simulink library "xblocks_library_pfbs"  (Simulink 7.6)
settings: Solver=ode45  SolverMode=SingleTasking  StartTime=0.0  StopTime=10.0  RelTol=1e-3
libraries: xbsIndex_r4 x369, monroe_library x47
(part 3 of 7)

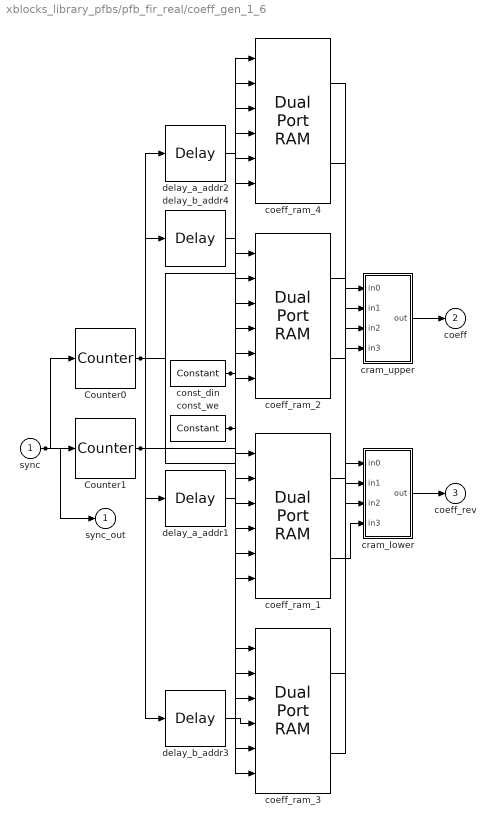
== system xblocks_library_pfbs/pfb_fir_real/coeff_gen_1_6 ==
  sync : Inport
  Counter0 : xbsIndex_r4/Counter  cnt_type=Free Running  cnt_to=Inf  operation=Up  start_count=8  cnt_by_val=1  arith_type=Unsigned  n_bits=11  bin_pt=0  load_pin=off  rst=on  en=off  explicit_period=on  period=1  dbl_ovrd=off  use_behavioral_HDL=off  implementation=Fabric  block_type=counter
  Counter1 : xbsIndex_r4/Counter  cnt_type=Free Running  cnt_to=Inf  operation=Down  start_count=2039  cnt_by_val=1  arith_type=Unsigned  n_bits=11  bin_pt=0  load_pin=off  rst=on  en=off  explicit_period=on  period=1  dbl_ovrd=off  use_behavioral_HDL=off  implementation=Fabric  block_type=counter
  coeff_ram_1 : xbsIndex_r4/Dual Port RAM  depth=2048  initVector=[-3.66227706703549e-006 -2.32001223055732e-005 -4.27476852292724e-005 -6.23051253222115e-005 -8.1872602220841e-005 -0.000101450275712516 -0.000121038305734028 -0.000140636852370183 -0.00016024607585228 -0.000179866136556684 -0.000199497195003349 -0.000219139411854352 -0.000238792947912406 -0.000258457964119436 -0.000278134621555034 -0.000297823081435025 -0.00031752350510998 -0.000337236054063722 -0.000356960889911885 -0.000376698174400365 -0.000396448069403875 -0.000416210736924445 -0.000435986339089932 -0.000455775038152512 -0.000475576996487234 -0.000495392376590451 -0.000515221341078369 -0.000535064052685532 -0.000554920674263309 -0.000574791368778434 -0.000594676299311432 -0.000614575629055151 -0.000634489521313247 -0.000654418139498664 -0.000674361647132113 -0.000694320207840599 -0.000714293985355835 -0.000734283143512765 -0.000754287846248034 -0.000774308257598449 -0.000794344541699504 -0.000814396862783775 -0.000834465385179446 -0.00085455027330876 -0.000874651691686487 -0.000894769804918378 -0.000914904777699676 -0.000935056774813504 -0.000955225961129376 -0.000975412501601635 -0.00099561656126791 -0.00101583830524761 -0.00103607789874029 -0.00105633550702419 -0.00107661129545462 -0.00109690542946247 -0.00111721807455258 -0.00113754939630225 -0.00115789956035966 -0.00117826873244228 -0.00119865707833536 -0.00121906476389031 -0.00123949195502323 -0.00125993881771322 -0.00128040551800089 -0.00130089222198679 -0.00132139909582981 -0.00134192630574561 -0.00136247401800508 -0.00138304239893273 -0.0014036316149051 -0.00142424183234923 -0.00144487321774102 -0.00146552593760373 -0.0014862001585063 -0.00150689604706182 -0.00152761376992592 -0.00154835349379522 -0.00156911538540568 -0.00158989961153107 -0.00161070633898134 -0.00163153573460101 -0.00165238796526762 -0.00167326319789008 -0.00169416159940713 -0.00171508333678569 -0.00173602857701927 -0.00175699748712639 -0.00177799023414891 -0.00179900698515051 -0.00182004790721505 -0.0018411131674449 -0.00186220293295942 -0.00188331737089327 -0.00190445664839487 -0.00192562093262472 -0.00194681039075383 -0.00196802518996205 -0.00198926549743652 -0.00201053148036997 -0.00203182330595915 -0.00205314114140324 -0.0020744851539021 -0.00209585551065479 -0.00211725237885783 -0.00213867592570362 -0.00216012631837886 -0.00218160372406278 -0.00220310830992565 -0.00222464024312707 -0.00224619969081432 -0.00226778682012079 -0.00228940179816431 -0.00231104479204548 -0.00233271596884606 -0.00235441549562733 -0.00237614353942842 -0.00239790026726473 -0.00241968584612619 -0.0024415004429757 -0.00246334422474741 -0.00248521735834514 -0.00250712001064065 -0.0025290523484721 -0.00255101453864227 -0.00257300674791699 -0.00259502914302347 -0.00261708189064861 -0.0026391651574374 -0.00266127910999121 -0.00268342391486616 -0.00270559973857143 -0.00272780674756764 -0.00275004510826513 -0.0027723149870224 -0.00279461655014431 -0.00281694996388051 -0.00283931539442373 -0.00286171300790811 -0.0028841429704076 -0.00290660544793418 -0.00292910060643627 -0.00295162861179701 -0.00297418962983265 -0.00299678382629077 -0.00301941136684874 -0.00304207241711193 -0.00306476714261208 -0.00308749570880561 -0.00311025828107197 -0.00313305502471193 -0.0031558861049459 -0.00317875168691227 -0.00320165193566569 -0.00322458701617542 -0.00324755709332363 -0.00327056233190375 -0.00329360289661871 -0.00331667895207931 -0.00333979066280252 -0.00336293819320978 -0.00338612170762535 -0.00340934137027454 -0.0034325973452821 -0.00345588979667048 -0.00347921888835816 -0.00350258478415793 -0.00352598764777525 -0.00354942764280647 -0.00357290493273721 -0.00359641968094064 -0.00361997205067573 -0.00364356220508568 -0.00366719030719606 -0.00369085651991323 -0.00371456100602259 -0.00373830392818688 -0.00376208544894448 -0.00378590573070776 -0.00380976493576126 -0.0038336632262601 -0.00385760076422821 -0.00388157771155665 -0.00390559423000192 -0.00392965048118421 -0.0039537466265857 -0.0039778828275489 -0.0040020592452749 ...(+37226 chars)]  distributed_mem=Block RAM  init_a=0  init_b=0  rst_a=off  rst_b=off  en_a=off  en_b=off  latency=2  write_mode_A=No Read On Write  write_mode_B=No Read On Write  dbl_ovrd=off  optimize=Area  use_rpm=on  block_type=dpram
  coeff_ram_2 : xbsIndex_r4/Dual Port RAM  depth=2048  initVector=[4.94480501293789e-005 0.000313528515560473 0.000578211328821063 0.000843496748818215 0.00110938503293764 0.00137587643704166 0.00164297121546728 0.00191066962102343 0.00217897190498901 0.00244787831711094 0.00271738910560136 0.00298750451713606 0.00325822479685175 0.0035295501883441 0.00380148093366576 0.00407401727332372 0.00434715944627736 0.00462090768993652 0.00489526224015883 0.00517022333124779 0.00544579119595085 0.00572196606545669 0.00599874816939369 0.00627613773582724 0.00655413499125781 0.00683274016061908 0.00711195346727528 0.00739177513301934 0.00767220537807098 0.00795324442107411 0.00823489247909495 0.00851714976762013 0.0088000165005541 0.00908349289021755 0.00936757914734485 0.00965227548108216 0.00993758209898553 0.0102234992070184 0.0105100270095498 0.0107971657093523 0.0110849155075997 0.0113732766038651 0.0116622491961191 0.0119518334807271 0.012242029652448 0.0125328379044316 0.0128242584282165 0.0131162914137289 0.0134089370492794 0.0137021955215617 0.0139960670156506 0.0142905517149995 0.0145856498014388 0.014881361455174 0.0151776868547828 0.0154746261772146 0.015772179597787 0.0160703472901847 0.0163691294264574 0.0166685261770175 0.0169685377106383 0.0172691641944524 0.0175704057939489 0.0178722626729722 0.0181747349937197 0.01847782291674 0.0187815266009308 0.019085846203537 0.0193907818801487 0.0196963337846997 0.0200025020694647 0.0203092868850582 0.0206166883804326 0.0209247067028753 0.0212333419980079 0.0215425944097839 0.0218524640804866 0.0221629511507274 0.0224740557594439 0.0227857780438981 0.0230981181396744 0.0234110761806776 0.0237246522991314 0.0240388466255762 0.0243536592888676 0.0246690904161739 0.0249851401329752 0.0253018085630606 0.0256190958285271 0.0259370020497773 0.0262555273455178 0.0265746718327575 0.0268944356268053 0.0272148188412687 0.0275358215880523 0.0278574439773549 0.028179686117669 0.0285025481157782 0.0288260300767556 0.0291501321039621 0.0294748542990447 0.0298001967619343 0.0301261595908447 0.0304527428822702 0.0307799467309838 0.0311077712300362 0.0314362164707532 0.0317652825427343 0.0320949695338515 0.0324252775302463 0.0327562066163295 0.0330877568747784 0.0334199283865353 0.0337527212308062 0.0340861354850587 0.0344201712250205 0.0347548285246777 0.0350901074562729 0.0354260080903038 0.0357625304955216 0.0360996747389289 0.0364374408857786 0.0367758289995716 0.0371148391420557 0.0374544713732239 0.0377947257513124 0.0381356023327992 0.0384771011724027 0.0388192223230798 0.0391619658360239 0.0395053317606644 0.0398493201446639 0.0401939310339176 0.0405391644725507 0.0408850205029176 0.0412314991656002 0.0415786004994061 0.0419263245413669 0.0422746713267372 0.0426236408889926 0.0429732332598279 0.0433234484691565 0.0436742865451078 0.0440257475140263 0.0443778314004699 0.0447305382272082 0.0450838680152215 0.0454378207836985 0.0457923965500355 0.0461475953298346 0.0465034171369023 0.0468598619832475 0.0472169298790813 0.0475746208328137 0.047932934851054 0.0482918719386078 0.0486514320984764 0.0490116153318553 0.0493724216381323 0.0497338510148863 0.0500959034578864 0.0504585789610893 0.0508218775166389 0.0511857991148646 0.0515503437442794 0.0519155113915794 0.0522813020416415 0.0526477156775226 0.053014752280458 0.0533824118298599 0.0537506943033161 0.0541195996765889 0.0544891279236135 0.0548592790164963 0.0552300529255142 0.0556014496191129 0.0559734690639055 0.0563461112246712 0.0567193760643543 0.0570932635440623 0.0574677736230651 0.0578429062587933 0.0582186614068372 0.0585950390209453 0.058972039053023 0.0593496614531316 0.0597279061694864 0.0601067731484563 0.0604862623345617 0.0608663736704737 0.0612471070970128 0.0616284625531474 0.0620104399759927 0.0623930393008099 0.0627762604610041 0.0631601033881235 0.0635445680118587 0.0639296542600405 0.0643153620586393 0.064701691331764 0.0650886420016601 0.0654762139887096 0.0658644072114286 0.0662532215864671 0.0666426570286074 0.0670327134507629 0.067423390763977 0.0678146888774221 0.0682066076983981 ...(+32980 chars)]  distributed_mem=Block RAM  init_a=0  init_b=0  rst_a=off  rst_b=off  en_a=off  en_b=off  latency=2  write_mode_A=No Read On Write  write_mode_B=No Read On Write  dbl_ovrd=off  optimize=Area  use_rpm=on  block_type=dpram
  coeff_ram_3 : xbsIndex_r4/Dual Port RAM  depth=2048  initVector=[0.999999981455428 0.999999256156816 0.9999974758801 0.999994640629567 0.999990750412045 0.9999858052369 0.999979805116038 0.999972750063907 0.999964640097494 0.999955475236325 0.999945255502468 0.99993398092053 0.999921651517657 0.999908267323534 0.999893828370388 0.999878334692983 0.999861786328625 0.999844183317156 0.99982552570096 0.999805813524958 0.99978504683661 0.999763225685917 0.999740350125415 0.99971642021018 0.999691435997827 0.999665397548507 0.999638304924911 0.999610158192265 0.999580957418334 0.999550702673419 0.99951939403036 0.999487031564532 0.999453615353845 0.999419145478749 0.999383622022225 0.999347045069795 0.999309414709511 0.999270731031964 0.999230994130277 0.99919020410011 0.999148361039656 0.99910546504964 0.999061516233323 0.999016514696497 0.99897046054749 0.998923353897159 0.998875194858894 0.998825983548619 0.998775720084785 0.998724404588377 0.998672037182911 0.998618617994431 0.998564147151511 0.998508624785256 0.998452051029298 0.998394426019799 0.998335749895448 0.998276022797461 0.998215244869582 0.998153416258081 0.998090537111756 0.998026607581926 0.997961627822441 0.997895597989672 0.997828518242513 0.997760388742386 0.997691209653232 0.997620981141516 0.997549703376226 0.997477376528869 0.997404000773475 0.997329576286594 0.997254103247294 0.997177581837164 0.997100012240311 0.997021394643359 0.996941729235451 0.996861016208246 0.996779255755918 0.996696448075158 0.996612593365171 0.996527691827675 0.996441743666904 0.996354749089604 0.99626670830503 0.996177621524954 0.996087488963654 0.995996310837921 0.995904087367053 0.995810818772859 0.995716505279653 0.995621147114259 0.995524744506007 0.995427297686731 0.99532880689077 0.995229272354969 0.995128694318676 0.995027073023739 0.994924408714512 0.994820701637845 0.994715952043093 0.994610160182107 0.994503326309239 0.994395450681337 0.994286533557745 0.994176575200305 0.994065575873355 0.993953535843724 0.993840455380737 0.99372633475621 0.993611174244453 0.993494974122263 0.993377734668931 0.993259456166233 0.993140138898437 0.993019783152294 0.992898389217045 0.992775957384412 0.992652487948607 0.992527981206318 0.992402437456722 0.992275857001473 0.992148240144707 0.99201958719304 0.991889898455565 0.991759174243852 0.99162741487195 0.99149462065638 0.991360791916138 0.991225928972696 0.991090032149994 0.990953101774447 0.990815138174937 0.990676141682815 0.990536112631903 0.990395051358487 0.990252958201319 0.990109833501616 0.989965677603059 0.98982049085179 0.989674273596413 0.989527026187993 0.989378748980052 0.98922944232857 0.989079106591985 0.98892774213119 0.98877534930953 0.988621928492808 0.988467480049272 0.988312004349628 0.988155501767025 0.987997972677064 0.987839417457792 0.987679836489702 0.98751923015573 0.987357598841259 0.987194942934109 0.987031262824544 0.986866558905266 0.986700831571417 0.986534081220575 0.986366308252751 0.986197513070394 0.986027696078385 0.985856857684035 0.985684998297086 0.985512118329711 0.985338218196507 0.9851632983145 0.984987359103141 0.984810400984302 0.984632424382279 0.984453429723789 0.984273417437968 0.984092387956369 0.983910341712962 0.983727279144134 0.983543200688683 0.983358106787821 0.983171997885169 0.98298487442676 0.982796736861033 0.982607585638834 0.982417421213414 0.982226244040427 0.982034054577931 0.981840853286381 0.981646640628634 0.981451417069944 0.98125518307796 0.981057939122726 0.980859685676679 0.980660423214647 0.980460152213848 0.980258873153888 0.980056586516761 0.979853292786845 0.979648992450902 0.979443685998075 0.979237373919888 0.979030056710245 0.978821734865424 0.978612408884082 0.978402079267248 0.978190746518324 0.977978411143081 0.977765073649662 0.977550734548574 0.977335394352693 0.977119053577255 0.976901712739862 0.976683372360474 0.976464032961412 0.976243695067352 0.976022359205328 0.975800025904726 0.975576695697283 0.97535236911709 0.975127046700582 0.974900728986545 0.974673416516108 0.974445109832743 0.974215809482264 ...(+32976 chars)]  distributed_mem=Block RAM  init_a=0  init_b=0  rst_a=off  rst_b=off  en_a=off  en_b=off  latency=2  write_mode_A=No Read On Write  write_mode_B=No Read On Write  dbl_ovrd=off  optimize=Area  use_rpm=on  block_type=dpram
  coeff_ram_4 : xbsIndex_r4/Dual Port RAM  depth=2048  initVector=[-4.94268847123748e-005 -0.000312679547413951 -0.000575330483273145 -0.000837379956314323 -0.00109882823207295 -0.00135967557759355 -0.00161992226142772 -0.00187956855363133 -0.0021386147257626 -0.00239706105087993 -0.0026549078035392 -0.00291215525979204 -0.00316880369718303 -0.00342485339474766 -0.00368030463301021 -0.00393515769398109 -0.00418941286115467 -0.00444307041950728 -0.00469613065549441 -0.00494859385704863 -0.0052004603135775 -0.00545173031596073 -0.00570240415654846 -0.0059524821291584 -0.00620196452907371 -0.00645085165304092 -0.00669914379926711 -0.00694684126741781 -0.00719394435861485 -0.00744045337543361 -0.00768636862190083 -0.00793169040349252 -0.00817641902713103 -0.00842055480118332 -0.00866409803545804 -0.00890704904120341 -0.009149408131105 -0.00939117561928297 -0.00963235182128986 -0.00987293705410845 -0.0101129316361489 -0.0103523358872466 -0.0105911501286599 -0.0108293746830673 -0.0110670098745656 -0.011304056028667 -0.0115405134722968 -0.0117763825337911 -0.0120116635428944 -0.0122463568307569 -0.0124804627299325 -0.0127139815743758 -0.0129469136994401 -0.013179259441875 -0.0134110191398235 -0.0136421931328201 -0.0138727817617878 -0.014102785369036 -0.0143322042982581 -0.0145610388945288 -0.0147892895043014 -0.0150169564754062 -0.0152440401570472 -0.0154705408997995 -0.015696459055608 -0.0159217949777833 -0.0161465490210007 -0.0163707215412965 -0.0165943128960663 -0.0168173234440621 -0.01703975354539 -0.0172616035615076 -0.0174828738552214 -0.0177035647906846 -0.017923676733394 -0.0181432100501883 -0.0183621651092446 -0.0185805422800769 -0.0187983419335326 -0.0190155644417906 -0.0192322101783587 -0.0194482795180707 -0.0196637728370842 -0.019878690512878 -0.0200930329242494 -0.0203068004513116 -0.0205199934754914 -0.0207326123795266 -0.0209446575474632 -0.0211561293646529 -0.0213670282177507 -0.0215773544947122 -0.0217871085847911 -0.0219962908785363 -0.0222049017677899 -0.0224129416456841 -0.0226204109066386 -0.0228273099463587 -0.0230336391618317 -0.0232393989513251 -0.0234445897143835 -0.0236492118518261 -0.0238532657657446 -0.0240567518594996 -0.0242596705377188 -0.0244620222062943 -0.0246638072723795 -0.0248650261443867 -0.0250656792319849 -0.0252657669460965 -0.0254652896988951 -0.0256642479038026 -0.0258626419754869 -0.0260604723298588 -0.0262577393840698 -0.0264544435565091 -0.0266505852668011 -0.0268461649358029 -0.0270411829856012 -0.0272356398395102 -0.0274295359220684 -0.0276228716590364 -0.0278156474773938 -0.0280078638053369 -0.0281995210722757 -0.0283906197088316 -0.0285811601468343 -0.0287711428193194 -0.0289605681605255 -0.0291494366058919 -0.0293377485920554 -0.0295255045568479 -0.0297127049392937 -0.0298993501796068 -0.0300854407191879 -0.0302709770006222 -0.0304559594676763 -0.0306403885652956 -0.0308242647396016 -0.0310075884378893 -0.0311903601086241 -0.0313725802014397 -0.0315542491671346 -0.0317353674576702 -0.0319159355261673 -0.0320959538269039 -0.0322754228153123 -0.0324543429479762 -0.0326327146826282 -0.0328105384781471 -0.0329878147945548 -0.0331645440930136 -0.0333407268358242 -0.0335163634864218 -0.0336914545093743 -0.0338660003703788 -0.0340400015362594 -0.0342134584749643 -0.0343863716555627 -0.0345587415482424 -0.0347305686243071 -0.0349018533561732 -0.0350725962173673 -0.0352427976825237 -0.0354124582273808 -0.0355815783287793 -0.0357501584646588 -0.0359181991140549 -0.0360857007570972 -0.0362526638750054 -0.0364190889500875 -0.0365849764657365 -0.0367503269064276 -0.0369151407577155 -0.0370794185062317 -0.0372431606396815 -0.0374063676468414 -0.0375690400175561 -0.0377311782427355 -0.0378927828143527 -0.0380538542254401 -0.0382143929700874 -0.0383743995434385 -0.0385338744416886 -0.0386928181620813 -0.0388512312029062 -0.0390091140634957 -0.0391664672442222 -0.0393232912464953 -0.0394795865727592 -0.0396353537264895 -0.0397905932121904 -0.0399453055353924 -0.0400994912026486 -0.0402531507215326 -0.0404062846006352 -0.0405588933495617 -0.0407109774789291 ...(+37258 chars)]  distributed_mem=Block RAM  init_a=0  init_b=0  rst_a=off  rst_b=off  en_a=off  en_b=off  latency=2  write_mode_A=No Read On Write  write_mode_B=No Read On Write  dbl_ovrd=off  optimize=Area  use_rpm=on  block_type=dpram
  const_din : xbsIndex_r4/Constant  const=0  gui_display_data_type=Fixed-point  arith_type=Signed (2's comp)  n_bits=18  bin_pt=17  preci_type=Single  exp_width=8  frac_width=24  explicit_period=on  period=1  equ=P=C  opselect=C  inp2=PCIN>>17  opr=+  inp1=P  carry=CIN  dbl_ovrd=off  block_type=constant
  const_we : xbsIndex_r4/Constant  const=0  gui_display_data_type=Fixed-point  arith_type=Boolean  n_bits=16  bin_pt=14  preci_type=Single  exp_width=8  frac_width=24  explicit_period=on  period=1  equ=P=C  opselect=C  inp2=PCIN>>17  opr=+  inp1=P  carry=CIN  dbl_ovrd=off  block_type=constant
  cram_lower : Subsystem
  cram_upper : Subsystem
  delay_a_addr1 : xbsIndex_r4/Delay  rst=off  infoeditControl=Selection of Reset will increase slice count due to use of real FFs and instead of SRLs  en=off  latency=2  dbl_ovrd=off  reg_retiming=off  block_type=delay
  delay_a_addr2 : xbsIndex_r4/Delay  rst=off  infoeditControl=Selection of Reset will increase slice count due to use of real FFs and instead of SRLs  en=off  latency=1  dbl_ovrd=off  reg_retiming=off  block_type=delay
  delay_b_addr3 : xbsIndex_r4/Delay  rst=off  infoeditControl=Selection of Reset will increase slice count due to use of real FFs and instead of SRLs  en=off  latency=1  dbl_ovrd=off  reg_retiming=off  block_type=delay
  delay_b_addr4 : xbsIndex_r4/Delay  rst=off  infoeditControl=Selection of Reset will increase slice count due to use of real FFs and instead of SRLs  en=off  latency=2  dbl_ovrd=off  reg_retiming=off  block_type=delay
  sync_out : Outport
  coeff : Outport  Port=2
  coeff_rev : Outport  Port=3
  wires:
  sync/1 -> Counter1/1, Counter0/1, sync_out/1
  Counter0/1 -> coeff_ram_4/1, coeff_ram_3/1, delay_a_addr2/1, delay_a_addr1/1
  const_din/1 -> coeff_ram_4/5, coeff_ram_4/2, coeff_ram_3/5, coeff_ram_3/2, coeff_ram_2/5, coeff_ram_2/2, coeff_ram_1/5, coeff_ram_1/2
  const_we/1 -> coeff_ram_4/6, coeff_ram_4/3, coeff_ram_3/6, coeff_ram_3/3, coeff_ram_2/6, coeff_ram_2/3, coeff_ram_1/6, coeff_ram_1/3
  Counter1/1 -> delay_b_addr4/1, delay_b_addr3/1, coeff_ram_2/4, coeff_ram_1/4
  cram_lower/1(out) -> coeff_rev/1
  cram_upper/1(out) -> coeff/1
  coeff_ram_1/2 -> cram_lower/4(in3)
  coeff_ram_2/2 -> cram_lower/3(in2)
  coeff_ram_3/2 -> cram_lower/2(in1)
  coeff_ram_4/2 -> cram_lower/1(in0)
  coeff_ram_4/1 -> cram_upper/4(in3)
  coeff_ram_3/1 -> cram_upper/3(in2)
  coeff_ram_2/1 -> cram_upper/2(in1)
  coeff_ram_1/1 -> cram_upper/1(in0)
  delay_b_addr4/1 -> coeff_ram_4/4
  delay_b_addr3/1 -> coeff_ram_3/4
  delay_a_addr2/1 -> coeff_ram_2/1
  delay_a_addr1/1 -> coeff_ram_1/1
